simulink model "Pendule"  (Simulink 7.2)
settings: Solver=ode45  StartTime=0.0  StopTime=30  RelTol=1e-3
values from neighbouring files (symbols this model uses):
  A = [0 0 1 0 ... (first row only)    [ChgmentBase13.m]    (also in CommObs14.m; ModelLin12.m = [0 0 1 0;0 0 0 1; 0 -(m/M)*g 0 0;0 (M+m)*g/(M*l) 0 0]; Stabilite15.m)
  B = [0 0 1/M -1/(M*l)]'    [ChgmentBase13.m]    (also in CommObs14.m; ModelLin12.m = [0 0 1/M -1/(M*l);0 0 0 0;0 0 0 0;0 0 0 0]; Stabilite15.m)
  C = [1 0 0 0 ... (first row only)    [ChgmentBase13.m]    (also in CommObs14.m; ModelLin12.m = [1 0 0 0;0 1 0 0;0 0 1 0;0 0 0 1]; Stabilite15.m)
  K = [0 k1 0 k2]    [ModelLin12.m]    (also in Stabilite15.m = acker(A,B,P))
undefined symbols (not defined in the file or in its folder): D
settings Model: Creator=Johnny  LastModifiedBy=Johnny

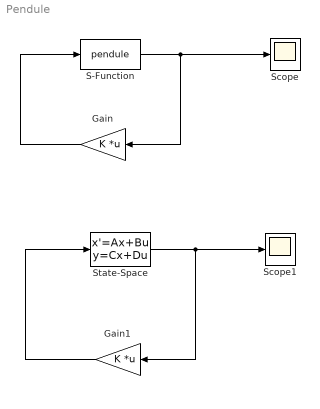
== system Pendule ==
  Gain : Gain  Orientation=left  Gain=K  Multiplication=Matrix(K*u)  ParameterDataType=sfix(16)  ParameterScaling=2^0  OutDataType=sfix(16)  OutScaling=2^0
  Gain1 : Gain  Orientation=left  Gain=K  Multiplication=Matrix(K*u)  ParameterDataType=sfix(16)  ParameterScaling=2^0  OutDataType=sfix(16)  OutScaling=2^0
  S-Function : S-Function  FunctionName=pendule  EnableBusSupport=off
  Scope : Scope
  Scope1 : Scope
  State-Space : StateSpace  A=A  B=B  C=C  D=D  X0=[2; pi/36 ; 0; 0]
  wires:
  Gain/1 -> S-Function/1
  S-Function/1 -> Scope/1, Gain/1
  Gain1/1 -> State-Space/1
  State-Space/1 -> Scope1/1, Gain1/1
